simulink model "ProportionalGainController_NO_ESTIMATOR_project"  (R2025b)
settings: Solver=FixedStepAuto  StartTime=0.0  StopTime=2  FixedStep=0.05  RelTol=1e-3
values from neighbouring files (symbols this model uses):
  A_b = [0 1 0 0; num21_a/Z num22_a/(R*Z) 0 num24_a/(R*r*Z) ; 0 0 0 1; num41_a/Z num42_a/(R*Z) 0 num44_a/(R*Z)]    [Project.m]    (also in Project_Jayce.m = double(vpa(A_b,14)); Project_template.m = [])
  B_b = [0; num2_b/den1_b ; 0; num4_b/den1_b]    [Project.m]    (also in Project_Jayce.m = double(vpa(B_b,14)); Project_template.m = [])
  D_b = [0; 0; 0; 0]    [Project.m]    (also in Project_Jayce.m = [0;0;0;0]; Project_template.m = [])
  K_pg = KLQR    [Project_Jayce.m]
settings Model: Creator=jboar  LastModifiedBy=jboar
settings DataIOCC: ReturnWorkspaceOutputs=off

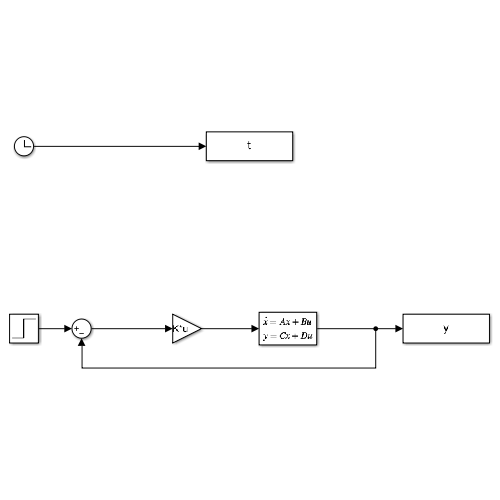
[thumbnail: Simulink's stored preview of the top-level diagram]
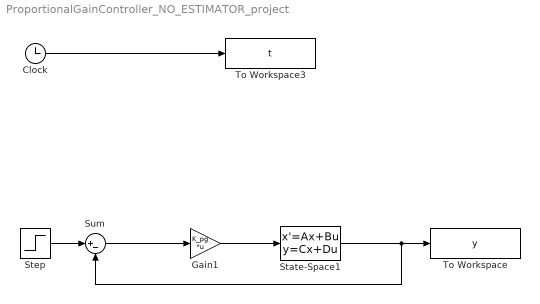
== system ProportionalGainController_NO_ESTIMATOR_project ==
  Clock : Clock
  Gain1 : Gain  Gain=K_pg  Multiplication=Matrix(K*u)
  State-Space1 : StateSpace  A=A_b  B=B_b  C=diag([1,1,1,1])  D=D_b  InitialCondition=0
  Step : Step  SampleTime=0
  Sum : Sum  Inputs=|+-
  To Workspace : ToWorkspace  VariableName=y  SampleTime=-1
  To Workspace3 : ToWorkspace  VariableName=t  SampleTime=-1
  wires:
  State-Space1/1 -> Sum/2, To Workspace/1
  Clock/1 -> To Workspace3/1
  Step/1 -> Sum/1
  Sum/1 -> Gain1/1
  Gain1/1 -> State-Space1/1
